simulink model "modelo"  (R2025b)
settings: Solver=VariableStepAuto  StartTime=0.0  StopTime=10  RelTol=1e-3
values from neighbouring files (symbols this model uses):
  Ue = [0.05; -1.17391; 0; 0]    [equilibrium.m]    (also in trim_vector.mat = [0.05 -1.17391 0 0])
undefined symbols (not defined in the file or in its folder): sigbuilder_block
settings Model: Creator=anade

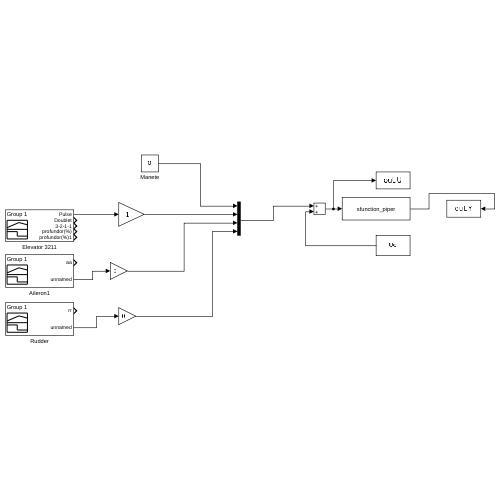
[thumbnail: Simulink's stored preview of the top-level diagram]
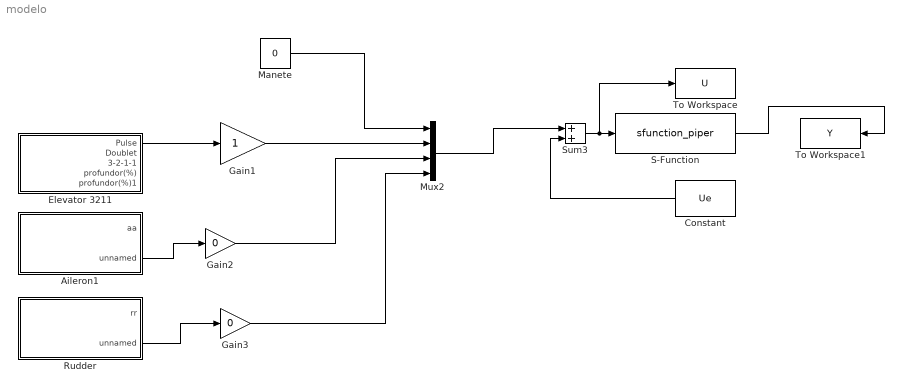
== system modelo ==
  Aileron1 : Subsystem  Tag=STV Subsys  LoadFcn=sigbuilder_block('load');  StartFcn=sigbuilder_block('start');  StopFcn=sigbuilder_block('stop');  ClipboardFcn=sigbuilder_block('clipboard');  mask(Sigbuilder block){tuvar=[0:10]}
      mask help: Simulink:masks:SigbuilderBlock_MD
      mask init:
      | if ~strcmp(get_param(bdroot(gcbh),'SimulationStatus'),'stopped') tuvar = sigbuilder_block('maskInit'); end
      settings: CopyFcn=sigbuilder_block('copy');  DeleteFcn=sigbuilder_block('delete');  ModelCloseFcn=sigbuilder_block('modelClose');  PreSaveFcn=sigbuilder_block('preSave');  PauseFcn=sigbuilder_block('pause');  ContinueFcn=sigbuilder_block('continue');  NameChangeFcn=sigbuilder_block('namechange');  OpenFcn=sigbuilder_block('open',[678.96 158.4 419.76 314.64 ]);  CloseFcn=sigbuilder_block('close');
      mask Display: plot(0, 0, 100, 100,[2, 2, 32, 32, 2], [68, 8, 8, 68, 68],[32, 2], [38, 38], [32, 19, 2],[53, 60, 44], [32, 17, 17, 2],[16, 16, 31, 31]);txt = getActiveGroup(gcbh);text(2, 100, txt,'verticalAlignment', 'top');
  Constant : Constant  Value=Ue
  Elevator 3211 : Subsystem  Tag=STV Subsys  LoadFcn=sigbuilder_block('load');  StartFcn=sigbuilder_block('start');  StopFcn=sigbuilder_block('stop');  ClipboardFcn=sigbuilder_block('clipboard');  mask(Sigbuilder block){tuvar=[0:10]}
      mask help: Simulink:masks:SigbuilderBlock_MD
      mask init:
      | if ~strcmp(get_param(bdroot(gcbh),'SimulationStatus'),'stopped') tuvar = sigbuilder_block('maskInit'); end
      settings: CopyFcn=sigbuilder_block('copy');  DeleteFcn=sigbuilder_block('delete');  ModelCloseFcn=sigbuilder_block('modelClose');  PreSaveFcn=sigbuilder_block('preSave');  PauseFcn=sigbuilder_block('pause');  ContinueFcn=sigbuilder_block('continue');  NameChangeFcn=sigbuilder_block('namechange');  OpenFcn=sigbuilder_block('open',[437.6 199.2 550.4 400 ]);  CloseFcn=sigbuilder_block('close');
      mask Display: plot(0, 0, 100, 100,[2, 2, 32, 32, 2], [68, 8, 8, 68, 68],[32, 2], [38, 38], [32, 19, 2],[53, 60, 44], [32, 17, 17, 2],[16, 16, 31, 31]);txt = getActiveGroup(gcbh);text(2, 100, txt,'verticalAlignment', 'top');
  Gain1 : Gain  OutDataTypeStr=double
  Gain2 : Gain  Gain=0
  Gain3 : Gain  Gain=0
  Manete : Constant  Value=0
  Mux2 : Mux
  Rudder : Subsystem  Tag=STV Subsys  LoadFcn=sigbuilder_block('load');  StartFcn=sigbuilder_block('start');  StopFcn=sigbuilder_block('stop');  ClipboardFcn=sigbuilder_block('clipboard');  mask(Sigbuilder block){tuvar=[0:10]}
      mask help: Simulink:masks:SigbuilderBlock_MD
      mask init:
      | if ~strcmp(get_param(bdroot(gcbh),'SimulationStatus'),'stopped') tuvar = sigbuilder_block('maskInit'); end
      settings: CopyFcn=sigbuilder_block('copy');  DeleteFcn=sigbuilder_block('delete');  ModelCloseFcn=sigbuilder_block('modelClose');  PreSaveFcn=sigbuilder_block('preSave');  PauseFcn=sigbuilder_block('pause');  ContinueFcn=sigbuilder_block('continue');  NameChangeFcn=sigbuilder_block('namechange');  OpenFcn=sigbuilder_block('open',[678.96 158.4 419.76 314.64 ]);  CloseFcn=sigbuilder_block('close');
      mask Display: plot(0, 0, 100, 100,[2, 2, 32, 32, 2], [68, 8, 8, 68, 68],[32, 2], [38, 38], [32, 19, 2],[53, 60, 44], [32, 17, 17, 2],[16, 16, 31, 31]);txt = getActiveGroup(gcbh);text(2, 100, txt,'verticalAlignment', 'top');
  S-Function : S-Function  FunctionName=sfunction_piper  Parameters=par_gen,par_aero,par_prop, Xe  SFunctionDeploymentMode=off  EnableBusSupport=off
  Sum3 : Sum
  To Workspace : ToWorkspace  VariableName=U  SaveFormat=Structure With Time  SampleTime=-1
  To Workspace1 : ToWorkspace  VariableName=Y  SaveFormat=Structure With Time  SampleTime=-1
  wires:
  S-Function/1 -> To Workspace1/1
  Sum3/1 -> To Workspace/1, S-Function/1
  Manete/1 -> Mux2/1
  Gain3/1 -> Mux2/4
  Gain1/1 -> Mux2/2
  Gain2/1 -> Mux2/3
  Elevator 3211/1(Pulse) -> Gain1/1
  Mux2/1 -> Sum3/1
  Constant/1 -> Sum3/2
  Aileron1/2(unnamed) -> Gain2/1
  Rudder/2(unnamed) -> Gain3/1

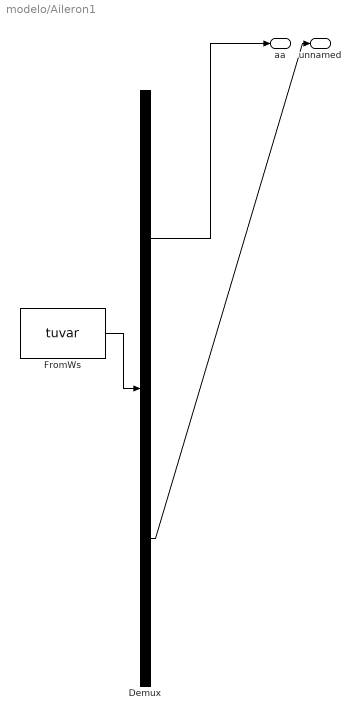
== system modelo/Aileron1 ==
  Demux : Demux  Tag=STV Demux  Outputs=2
      settings: DisplayOption=none
  FromWs : FromWorkspace  Tag=STV FromWs  VariableName=tuvar
      SigBuilderData=|
      | common.afterFinalStr = 'Extrapolate'
      | common.sampleTime = '0'
      | dataSet.timeRange = [0 100]
      | dataSet.name = 'Group 1'
      | sbobj.Groups.Name = 'Group 1'
      | sbobj.Groups.Signals(1).Name = 'aa'
      | sbobj.Groups.Signals(1).XData = [0 5 6 100]
      | sbobj.Groups.Signals(1).YData = [0 0 0 0]
      | sbobj.Groups.Signals(2).Name = 'unnamed'
      | sbobj.Groups.Signals(2).XData = [0 0.1 0.2 0.3 0.4 0.5 0.6 0.7 0.8 0.9 1 1.1 1.2 1.3 1.4 1.5 1.6 1.7 1.8 1.9 2 2.1 2.2 2.3 2.4 2.5 2.6 2.7 2.8 2.9 3 3.1 3.2 3.3 3.4 3.5 3.6 3.7 3.8 3.9 4 4.1 4.2 4.3 4.4 4.5 4.6 4.7 4.8 4.9 5 5.1 5.2 5.3 5.4 5.5 5.6 5.7 5.8 5.9 6 6.1 100]
      | sbobj.Groups.Signals(2).YData = [0.00221744081466 0.00217031692485 0.00212581102893 0.00208915911464 0.261799387799 0.261799387799 0.261799387799 0.261799387799 0.261799387799 0.261799387799 0.261799387799 0.261799387799 0.261799387799 0.261799387799 -0.261799387799 -0.261799387799 -0.261799387799 -0.261799387799 -0.261799387799 -0.261799387799 -0.261799387799 -0.261799387799 -0.261799387799 -0.261799387799 -0.194469821245 -0.0351936917018 0.00127496301858 0.00109955742876 0.00119642320224 -0.000992219679759 0.00182997772072 0.00157865030843 0.00340601003527 0.00134826684717 0.000777544181763 -0.00101578162466 0.00130376095124 0.00271485965148 0.00301854694132 0.00147131255943 0.00442179165993 0.00253160008002 0.00248709418409 0.00243997029429 0.00239546439836 0.00235357649631 0.00230645260651 0.00226456470446 0.00222005880854 0.00217817090649 0.0021415189922 0.0086236718341 -0.003282964323 -0.0168258466539 0.00552658507644 0.00425162205786 0.00273842159638 0.00219126087588 0.0020106192983 0.00196349540849 0.0019504054391 0.00192946148808 0.00192946148808]
      | sbobj.Groups.TimeRange = [0 100]
  aa : Outport  Tag=STV Outport
  unnamed : Outport  Tag=STV Outport  Port=2
  wires:
  FromWs/1 -> Demux/1
  Demux/1 -> aa/1
  Demux/2 -> unnamed/1

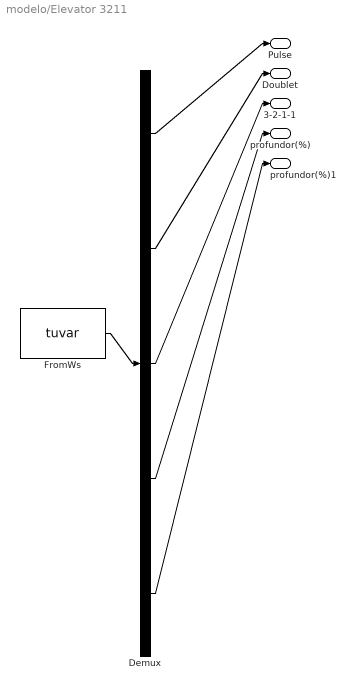
== system modelo/Elevator 3211 ==
  Demux : Demux  Tag=STV Demux  Outputs=5
      settings: DisplayOption=none
  FromWs : FromWorkspace  Tag=STV FromWs  VariableName=tuvar
      SigBuilderData=|
      | common.afterFinalStr = 'Extrapolate'
      | common.sampleTime = '0'
      | dataSet.timeRange = [0 100]
      | dataSet.name = 'Group 1'
      | sbobj.Groups.Name = 'Group 1'
      | sbobj.Groups.Signals(1).Name = 'Pulse'
      | sbobj.Groups.Signals(1).XData = [0 5 5 6 6 100]
      | sbobj.Groups.Signals(1).YData = [0 0 2 2 0 0]
      | sbobj.Groups.Signals(2).Name = 'Doublet'
      | sbobj.Groups.Signals(2).XData = [0 5 5 5.1 5.25 5.25 5.4 5.5 5.5 5.6 5.7 100]
      | sbobj.Groups.Signals(2).YData = [0 0 5 5 5 -5 -5 -5 0 0 0 0]
      | sbobj.Groups.Signals(3).Name = '3-2-1-1'
      | sbobj.Groups.Signals(3).XData = [0 5 5 5.1 5.2 5.3 5.3 5.4 5.5 5.5 5.6 5.6 5.7 5.7 100]
      | sbobj.Groups.Signals(3).YData = [0 0 3 3 3 3 -3 -3 -3 3 3 -3 -3 0 0]
      | sbobj.Groups.Signals(4).Name = 'profundor(%)'
      | sbobj.Groups.Signals(4).XData = [0 0.1 0.2 0.3 0.4 0.5 0.6 0.7 0.8 0.9 1 1.1 1.2 1.3 1.4 1.5 1.6 1.7 1.8 1.9 2 2.1 2.2 2.3 2.4 2.5 2.6 2.7 2.8 2.9 3 3.1 3.2 3.3 3.4 3.5 3.6 3.7 3.8 3.9 4 4.1 4.2 4.3 4.4 4.5 4.6 4.7 4.8 4.9 5 5.1 5.2 5.3 5.4 5.5 5.6 5.7 5.8 5.9 6 6.1 6.2 6.3 6.4 6.5 6.6 6.7 6.8 6.9 7 7.1 7.2 7.3 7.4 7.5 7.6 7.7 7.8 7.9 8 8.1 8.2 8.3 8.4 8.5 8.6 8.7 8.8 8.9 9 9.1 9.2 9.3 9.4 9.5 9.6 9.7 9.8 9.9 100]
      | sbobj.Groups.Signals(4).YData = [0.0196349540849 0.0196349540849 0.0196349540849 0.0194643599637 0.0116817814396 0.00765518966713 0.0169049757658 0.018891454736 0.0196349540849 0.0196349540849 0.0196349540849 0.0196349540849 0.0196349540849 0.0196349540849 0.0179523574034 0.0191731785037 0.0196349540849 0.0196349540849 0.0196349540849 0.0196349540849 0.0196349540849 0.0196349540849 0.0314787404534 0.0839220028003 0.198297815363 0.188959503412 0.0178814932476 -0.25870342875 -0.118169654383 0.0196349540849 0.0196349540849 0.0196349540849 0.0196349540849 0.0196349540849 0.0196349540849 0.0196349540849 0.0196349540849 0.0196349540849 0.0196349540849 0.0196349540849 0.0196349540849 0.0196349540849 0.0196349540849 0.0196349540849 0.0196349540849 0.0196349540849 0.0196349540849 0.0196349540849 0.0196349540849 0.0196349540849 0.0196349540849 0.0196349540849 0.0196349540849 0.0196349540849 0.0196349540849 0.0196349540849 0.0196349540849 0.0196349540849 0.0196349540849 0.0196349540849 0.0196349540849 0.0196349540849 0.0196349540849 0.0196349540849 0.0196349540849 0.0196349540849 0.0196349540849 0.0196349540849 0.0196349540849 0.0196349540849 0.0196349540849 0.0196349540849 0.0196349540849 0.0196349540849 0.0196349540849 0.0196349540849 0.0196349540849 0.0196349540849 0.0196349540849 0.0196349540849 0.0196349540849 0.0196349540849 0.0196349540849 0.0196349540849 0.0196349540849 0.0196349540849 0.0196349540849 0.0218905135147 0.0271099036102 0.0301069295969 0.0311266271794 0.0327616225817 0.0340801153602 0.0403792423468 0.0492883514228 0.051799395427 0.0504916604523 0.0493694755119 0.034098029423 0.0237390701567 0.0237390701567]
      | sbobj.Groups.Signals(5).Name = 'profundor(%)1'
      | sbobj.Groups.Signals(5).XData = [0 0.1 0.2 0.3 0.4 0.5 0.6 0.7 0.8 0.9 1 1.1 1.2 1.3 1.4 1.5 1.6 1.7 1.8 1.9 2 2.1 2.2 2.3 2.4 2.5 2.6 2.7 2.8 2.9 3 3.1 3.2 3.3 3.4 3.5 3.6 3.7 3.8 3.9 4 4.1 4.2 4.3 4.4 4.5 4.6 4.7 4.8 4.9 5 5.1 5.2 5.3 5.4 5.5 5.6 5.7 5.8 5.9 6 6.1 6.2 6.3 6.4 6.5 6.6 6.7 6.8 6.9 7 7.1 7.2 7.3 7.4 7.5 7.6 7.7 7.8 7.9 8 8.1 8.2 8.3 8.4 8.5 8.6 8.7 8.8 8.9 9 9.1 9.2 9.3 9.4 9.5 9.6 9.7 9.8 9.9 100]
      | sbobj.Groups.Signals(5).YData = [-0.054191556864 -0.0505032201968 -0.00531497341473 0.0155205476261 0.0181327033361 0.0196349540849 0.0196349540849 0.0196349540849 0.0196349540849 0.0196349540849 0.0196349540849 0.0196349540849 0.0196349540849 0.0196349540849 0.0410808928885 0.0754235175198 0.123271396562 0.196913068895 0.251200340827 0.116336824719 -0.0748264308208 -0.261799387799 -0.199433444343 -0.0757128197049 0.0196349540849 0.0196349540849 0.0196349540849 0.0196349540849 0.0196349540849 0.0196349540849 0.0196349540849 0.0196349540849 0.0196349540849 0.0196349540849 0.0196349540849 0.0196349540849 0.0196349540849 0.0196349540849 0.0196349540849 0.0196349540849 0.0196349540849 0.0196349540849 0.0196349540849 0.0196349540849 0.0196349540849 0.0196349540849 0.0196349540849 0.0196349540849 0.0196349540849 0.0196349540849 0.0196349540849 0.0196349540849 0.0196349540849 0.0196349540849 0.0196349540849 0.0196349540849 0.0196349540849 0.0196349540849 0.0196349540849 0.0196349540849 0.0196349540849 0.0196349540849 0.0196349540849 0.0196349540849 0.0196349540849 0.0196827866756 0.0226317750035 0.0255563589025 0.0292186688541 0.0422716330905 0.0523598775598 0.0523598775598 0.0523598775598 0.0509888702211 0.0473815171238 0.0438513974564 0.0433271256207 0.0410311116253 0.0364203319362 0.0309292771727 0.0237414383072 0.0196349540849 0.0196349540849 0.0196349540849 0.018119083107 0.0115684976614 0.00654498469498 0.000423923348124 0.00140538642808 0.0062795798446 0.00196349540849 0.00196349540849 0.00196349540849 0.00878991506599 0.017282810706 0.0189897911281 0.0194014098529 0.0225115859996 0.0447366939424 0.0545491175867 0.0545491175867]
      | sbobj.Groups.TimeRange = [0 100]
  Pulse : Outport  Tag=STV Outport
  Doublet : Outport  Tag=STV Outport  Port=2
  3-2-1-1 : Outport  Tag=STV Outport  Port=3
  profundor(%) : Outport  Tag=STV Outport  Port=4
  profundor(%)1 : Outport  Tag=STV Outport  Port=5
  wires:
  FromWs/1 -> Demux/1
  Demux/1 -> Pulse/1
  Demux/2 -> Doublet/1
  Demux/3 -> 3-2-1-1/1
  Demux/4 -> profundor(%)/1
  Demux/5 -> profundor(%)1/1

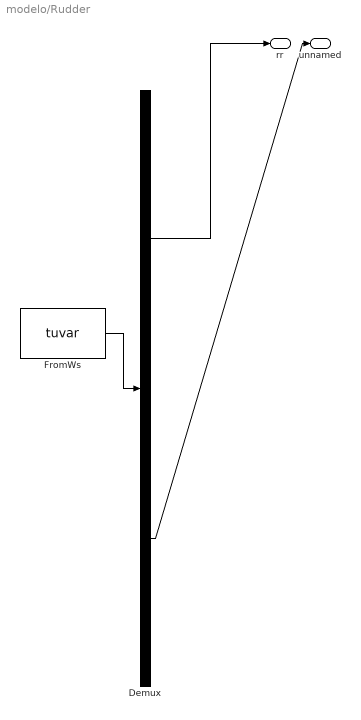
== system modelo/Rudder ==
  Demux : Demux  Tag=STV Demux  Outputs=2
      settings: DisplayOption=none
  FromWs : FromWorkspace  Tag=STV FromWs  VariableName=tuvar
      SigBuilderData=|
      | common.afterFinalStr = 'Extrapolate'
      | common.sampleTime = '0'
      | dataSet.timeRange = [0 100]
      | dataSet.name = 'Group 1'
      | sbobj.Groups.Name = 'Group 1'
      | sbobj.Groups.Signals(1).Name = 'rr'
      | sbobj.Groups.Signals(1).XData = [0 5 6 100]
      | sbobj.Groups.Signals(1).YData = [0 0 0 0]
      | sbobj.Groups.Signals(2).Name = 'unnamed'
      | sbobj.Groups.Signals(2).XData = [0 0.1 0.2 0.3 0.4 0.5 0.6 0.7 0.8 0.9 1 1.1 1.2 1.3 1.4 1.5 1.6 1.7 1.8 1.9 2 2.1 2.2 2.3 2.4 2.5 2.6 2.7 2.8 2.9 3 3.1 3.2 3.3 3.4 3.5 3.6 3.7 3.8 3.9 4 4.1 4.2 4.3 4.4 4.5 4.6 4.7 4.8 4.9 5 5.1 5.2 5.3 5.4 5.5 5.6 5.7 5.8 5.9 6 100]
      | sbobj.Groups.Signals(2).YData = [0.00608945376021 0.00609207175409 0.00609468974796 0.00608945376021 0.0210512887729 0.0370158154409 0.0237975643509 0.00421497014357 -0.014870205227 -0.0286303810497 -0.0367592520409 -0.0390787946168 -0.0338401888669 -0.0214649318057 0.00426209403337 0.0288110226273 0.0168494085988 -0.00520195383557 -0.0261485228534 -0.0398615747863 -0.0448828870443 -0.0425685804561 -0.0338846947628 -0.0209989288954 0.0198182136564 0.0228603225426 0.0177735604377 0.0154959057638 0.014697417631 0.0143204265126 0.0138884575227 0.0135585902941 0.0132679929737 0.012982631641 0.0127574841675 0.0124695048409 0.0122181774286 0.0119877939673 0.0117600284999 0.0115532069836 0.0113542394488 0.00691673982565 0.00695600973382 0.00699004365424 0.00701622359302 0.00703454955016 0.00704763951955 0.00705287550731 0.00705287550731 0.00704502152568 0.00703454955016 0.261799387799 0.261799387799 -0.261799387799 0.126027607293 0.063085798478 0.0223917016385 0.00996408469964 0.00673609824807 0.00654760268886 0.00664185046846 0.00664185046846]
      | sbobj.Groups.TimeRange = [0 100]
  rr : Outport  Tag=STV Outport
  unnamed : Outport  Tag=STV Outport  Port=2
  wires:
  FromWs/1 -> Demux/1
  Demux/1 -> rr/1
  Demux/2 -> unnamed/1
